simulink model "ControllerModel_sim_2020_HILS"  (R2020b)
settings: Solver=FixedStepAuto  StartTime=0.0  StopTime=Endtime  FixedStep=0.05  RelTol=1e-3  EnableMultiTasking=on
values from neighbouring files (symbols this model uses):
  Kd = 0    [ControllerModel_2020_HILS.m]
  Ki = 0.1    [ControllerModel_2020_HILS.m]
  Kp = 0.1    [ControllerModel_2020_HILS.m]
  SV = 1000    [ControllerModel_2020_HILS.m]
libraries: arduinolib x5
settings Model: SILPILModeSetting=veronly  ExtModeTrigDuration=2  Creator=005274  LastModifiedBy=005274
settings OptimizationCC: EnhancedBackFolding=on  PassReuseOutputArgsAs=Individual arguments  ZeroExternalMemoryAtStartup=off  ZeroInternalMemoryAtStartup=off  MaxStackSize=64  OptimizeBlockOrder=speed  DifferentSizesBufferReuse=on  OptimizationCustomize=off  EfficientTunableParamExpr=on
settings DebuggingCC: ParameterTunabilityLossMsg=error
settings HardwareCC: ProdBitPerInt=16  ProdBitPerPointer=16  ProdBitPerSizeT=16  ProdBitPerPtrDiffT=16  ProdLargestAtomicFloat=None  ProdWordSize=8  ProdHWDeviceType=Atmel->AVR  UseEmbeddedCoderFeatures=off  UseSimulinkCoderFeatures=off
settings SFSimCC: MATLABDynamicMemAlloc=off
settings RTWCC: Description=Embedded Coder  SystemTargetFile=ert.tlc  HardwareBoard=Arduino Mega 2560  TemplateMakefile=ert_default_tmf  Toolchain=Arduino AVR  BuildConfiguration=Faster Runs
settings CodeAppCC: ForceParamTrailComments=on  IgnoreCustomStorageClasses=off  OperatorAnnotations=on  SimulinkDataObjDesc=on  SFDataObjDesc=on  InsertBlockDesc=on
settings ERTTargetCC: SupportContinuousTime=on  SupportNonInlinedSFcns=on  SupportVariableSizeSignals=on  ExtModeStaticAllocSize=2048

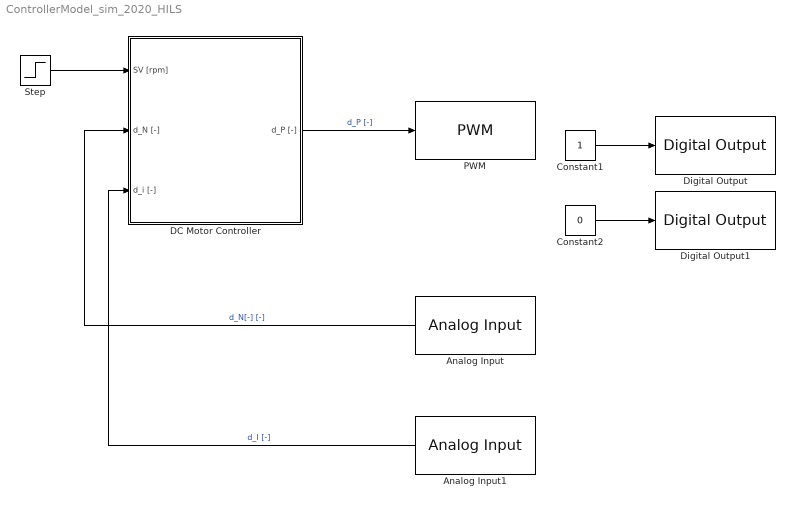
== system ControllerModel_sim_2020_HILS ==
  Analog Input : arduinolib/Analog Input  pinNumber=5  ReadResultsOnly=off  ConversionTriggerSource=Software  ExternalTriggerType=uint32( 0 )  OutputDataType=uint16  EnableConversionCompleteNotify=off  EnableOuputStatus=off  SampleTime=-1  blockPlatform=arduino
  Analog Input1 : arduinolib/Analog Input  pinNumber=8  ReadResultsOnly=off  ConversionTriggerSource=Software  ExternalTriggerType=uint32( 0 )  OutputDataType=uint16  EnableConversionCompleteNotify=off  EnableOuputStatus=off  SampleTime=-1  blockPlatform=arduino
  Constant1 : Constant
  Constant2 : Constant  Value=0
  DC Motor Controller : Subsystem
  Digital Output : arduinolib/Digital Output  pinNumber=8  Direction=output  blockPlatform=arduino
  Digital Output1 : arduinolib/Digital Output  pinNumber=7  Direction=output  blockPlatform=arduino
  PWM : arduinolib/PWM  pinNumber=10  frequencyType=Default  desiredFrequency=490.2  achievableFrequency=490.2
  Step : Step  After=SV  SampleTime=0
  wires:
  DC Motor Controller/1(d_P [-]) -> PWM/1  "d_P [-]"
  Analog Input/1 -> DC Motor Controller/2(d_N [-])  "d_N[-] [-]"
  Analog Input1/1 -> DC Motor Controller/3(d_i [-])  "d_I [-]"
  Step/1 -> DC Motor Controller/1(SV [rpm])
  Constant1/1 -> Digital Output/1
  Constant2/1 -> Digital Output1/1

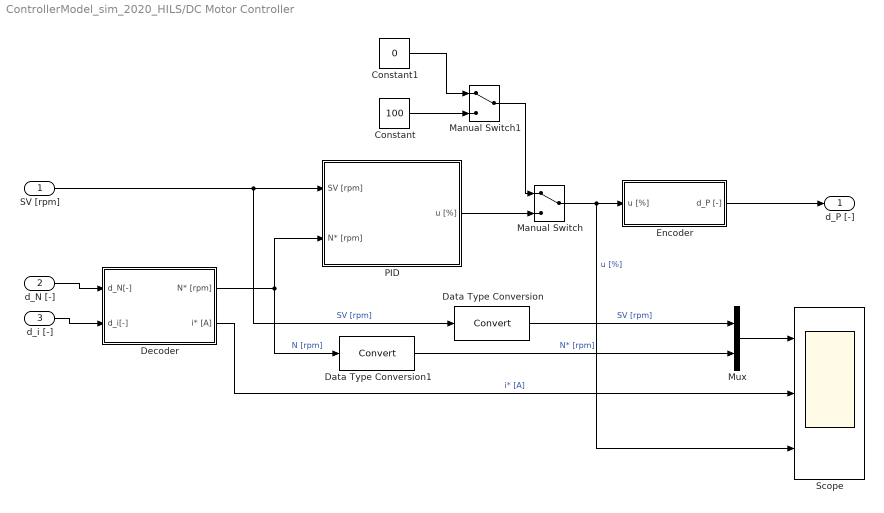
== system ControllerModel_sim_2020_HILS/DC Motor Controller ==
  SV [rpm] : Inport
  d_N [-] : Inport  Port=2
  d_i [-] : Inport  Port=3
  Constant : Constant  Value=100
  Constant1 : Constant  Value=0
  Data Type Conversion : DataTypeConversion
  Data Type Conversion1 : DataTypeConversion
  Decoder : Subsystem
  Encoder : Subsystem
  Manual Switch : ManualSwitch
  Manual Switch1 : ManualSwitch
  Mux : Mux  Inputs=2
  PID : Subsystem
  Scope : Scope  NumInputPorts=3
  d_P [-] : Outport
  wires:
  PID/1(u [%]) -> Manual Switch/2
  Decoder/2(i* [A]) -> Scope/2  "i* [A]"
  Decoder/1(N* [rpm]) -> PID/2(N* [rpm]), Data Type Conversion1/1  "N [rpm]"
  Constant1/1 -> Manual Switch1/1
  Manual Switch1/1 -> Manual Switch/1
  SV [rpm]/1 -> Data Type Conversion/1, PID/1(SV [rpm])  "SV [rpm]"
  Manual Switch/1 -> Scope/3, Encoder/1(u [%])  "u [%]"
  Encoder/1(d_P [-]) -> d_P [-]/1
  d_i [-]/1 -> Decoder/2(d_i[-])
  d_N [-]/1 -> Decoder/1(d_N[-])
  Mux/1 -> Scope/1
  Constant/1 -> Manual Switch1/2
  Data Type Conversion/1 -> Mux/1  "SV [rpm]"
  Data Type Conversion1/1 -> Mux/2  "N* [rpm]"

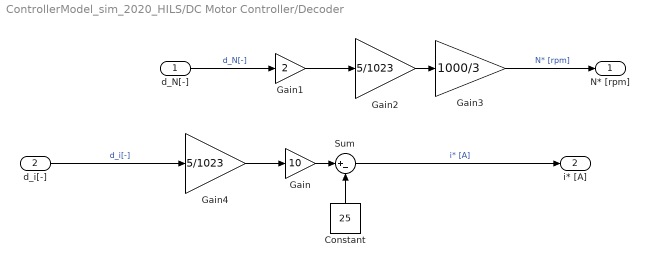
== system ControllerModel_sim_2020_HILS/DC Motor Controller/Decoder ==
  d_N[-] : Inport
  d_i[-] : Inport  Port=2
  Constant : Constant  Value=25
  Gain : Gain  Gain=10
  Gain1 : Gain  Gain=2
  Gain2 : Gain  Gain=5/1023
  Gain3 : Gain  Gain=1000/3
  Gain4 : Gain  Gain=5/1023
  Sum : Sum  Inputs=|+-
  N* [rpm] : Outport
  i* [A] : Outport  Port=2
  wires:
  Gain/1 -> Sum/1
  Constant/1 -> Sum/2
  d_i[-]/1 -> Gain4/1  "d_i[-]"
  Sum/1 -> i* [A]/1  "i* [A]"
  Gain1/1 -> Gain2/1
  d_N[-]/1 -> Gain1/1  "d_N[-]"
  Gain2/1 -> Gain3/1
  Gain3/1 -> N* [rpm]/1  "N* [rpm]"
  Gain4/1 -> Gain/1

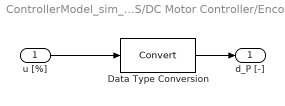
== system ControllerModel_sim_2020_HILS/DC Motor Controller/Encoder ==
  u [%] : Inport
  Data Type Conversion : DataTypeConversion
  d_P [-] : Outport
  wires:
  Data Type Conversion/1 -> d_P [-]/1
  u [%]/1 -> Data Type Conversion/1

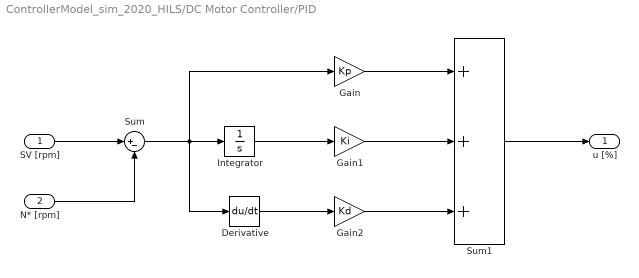
== system ControllerModel_sim_2020_HILS/DC Motor Controller/PID ==
  SV [rpm] : Inport
  N* [rpm] : Inport  Port=2
  Derivative : Derivative
  Gain : Gain  Gain=Kp
  Gain1 : Gain  Gain=Ki
  Gain2 : Gain  Gain=Kd
  Integrator : Integrator
  Sum : Sum  Inputs=|+-
  Sum1 : Sum  Inputs=+++
  u [%] : Outport
  wires:
  N* [rpm]/1 -> Sum/2
  SV [rpm]/1 -> Sum/1
  Sum/1 -> Derivative/1, Gain/1, Integrator/1
  Derivative/1 -> Gain2/1
  Integrator/1 -> Gain1/1
  Gain1/1 -> Sum1/2
  Gain/1 -> Sum1/1
  Gain2/1 -> Sum1/3
  Sum1/1 -> u [%]/1
